simulink model "ex5"  (Simulink 6.0)
settings: Solver=ode45  StartTime=0.0  StopTime=10.0  RelTol=1e-3
settings Model: LastModifiedBy=lxy

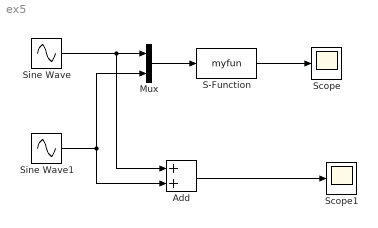
== system ex5 ==
  Add : Sum  OutScaling=2^-10
  Mux : Mux  Inputs=2
  S-Function : S-Function  FunctionName=myfun
  Scope : Scope
  Scope1 : Scope
  Sine Wave : Sin  Amplitude=2  SampleTime=0
  Sine Wave1 : Sin  Frequency=2  Phase=pi/2  SampleTime=0
  wires:
  Sine Wave/1 -> Mux/1, Add/1
  Sine Wave1/1 -> Mux/2, Add/2
  S-Function/1 -> Scope/1
  Mux/1 -> S-Function/1
  Add/1 -> Scope1/1
